simulink model "SynchGenerator_DQ_ThreePhaseFault"  (R2018a)
settings: Solver=FixedStepAuto  StartTime=0.0  StopTime=0.3  FixedStep=0.00005  MaxStep=200e-6  RelTol=1e-4  EnableMultiTasking=on
values from neighbouring files (symbols this model uses):
  fn = 60    [param_SynchGenerator_Kundur_3_1.m]    (also in param_SynchGenerator_Kundur_3_1_mathworks.m)
  ifn = 1300    [param_SynchGenerator_Kundur_3_1.m]    (also in param_SynchGenerator_Kundur_3_1_mathworks.m)
  Isbase = Pn/Vn/sqrt(3)*sqrt(2)    [param_SynchGenerator_Kundur_3_1.m]    (also in param_SynchGenerator_Kundur_3_1_mathworks.m)
  J = 2*H*Pn/wm^2    (= 28897.645918)    [param_SynchGenerator_Kundur_3_1.m]    (also in param_SynchGenerator_Kundur_3_1_mathworks.m)
  Ll = 0.4129e-3    (= 0.0004129)    [param_SynchGenerator_Kundur_3_1.m]    (also in param_SynchGenerator_Kundur_3_1_mathworks.m)
  Llfd = Llfd_pu*Lfbase    (= 0.0521181521186)    [param_SynchGenerator_Kundur_3_1.m]    (also in param_SynchGenerator_Kundur_3_1_mathworks.m)
  Llkd_pu = 0.1713    [param_SynchGenerator_Kundur_3_1.m]    (also in param_SynchGenerator_Kundur_3_1_mathworks.m)
  Llkq1_pu = 0.7252    [param_SynchGenerator_Kundur_3_1.m]    (also in param_SynchGenerator_Kundur_3_1_mathworks.m)
  Llkq2_pu = 0.125    [param_SynchGenerator_Kundur_3_1.m]    (also in param_SynchGenerator_Kundur_3_1_mathworks.m)
  Lmd = 4.5696e-3    (= 0.0045696)    [param_SynchGenerator_Kundur_3_1.m]    (also in param_SynchGenerator_Kundur_3_1_mathworks.m)
  Lmq = 4.432e-3    (= 0.004432)    [param_SynchGenerator_Kundur_3_1.m]    (also in param_SynchGenerator_Kundur_3_1_mathworks.m)
  Lsbase = Zsbase/wbase    (= 0.00275295036699)    [param_SynchGenerator_Kundur_3_1.m]    (also in param_SynchGenerator_Kundur_3_1_mathworks.m)
  Ns_Nf = 2/3*Ifbase/Isbase    [param_SynchGenerator_Kundur_3_1.m]    (also in param_SynchGenerator_Kundur_3_1_mathworks.m)
  Pn = 555e6    (= 555000000)    [param_SynchGenerator_Kundur_3_1.m]    (also in param_SynchGenerator_Kundur_3_1_mathworks.m)
  Rf = 0.0715    [param_SynchGenerator_Kundur_3_1.m]    (also in param_SynchGenerator_Kundur_3_1_mathworks.m)
  Rkd_pu = 0.0284    [param_SynchGenerator_Kundur_3_1.m]    (also in param_SynchGenerator_Kundur_3_1_mathworks.m)
  Rkq1_pu = 0.00619    [param_SynchGenerator_Kundur_3_1.m]    (also in param_SynchGenerator_Kundur_3_1_mathworks.m)
  Rkq2_pu = 0.02368    [param_SynchGenerator_Kundur_3_1.m]    (also in param_SynchGenerator_Kundur_3_1_mathworks.m)
  Rs = 0.0031    [param_SynchGenerator_Kundur_3_1.m]    (also in param_SynchGenerator_Kundur_3_1_mathworks.m)
  Vn = 24e3    (= 24000)    [param_SynchGenerator_Kundur_3_1.m]    (also in param_SynchGenerator_Kundur_3_1_mathworks.m)
  Vsbase = Vn/sqrt(3)*sqrt(2)    [param_SynchGenerator_Kundur_3_1.m]    (also in param_SynchGenerator_Kundur_3_1_mathworks.m)
  Zsbase = Vn^2/Pn    (= 1.03783783784)    [param_SynchGenerator_Kundur_3_1.m]    (also in param_SynchGenerator_Kundur_3_1_mathworks.m)
libraries: powerlib x9
Description:
  | Copyright 2008-2016 The MathWorks, Inc.
settings Model: Creator=MathWorks  LastModifiedBy=acs-mmi
settings DataIOCC: LimitDataPoints=on  SaveFormat=Array
settings OptimizationCC: ExpressionDepthLimit=2147483647  LifeSpan=inf
settings DebuggingCC: UnderspecifiedInitializationDetection=Classic  MergeDetectMultiDrivingBlocksExec=none  SolverPrmCheckMsg=warning  UnconnectedInputMsg=none  UnconnectedOutputMsg=none  UnconnectedLineMsg=none  StateNameClashWarn=warning  SFUnexpectedBacktrackingDiag=warning  SFNoUnconditionalDefaultTransitionDiag=warning  SFExecutionAtInitializationDiag=none
settings HardwareCC: ProdBitPerPointer=32  ProdBitPerSizeT=32  ProdBitPerPtrDiffT=32  ProdLargestAtomicFloat=None  ProdIntDivRoundTo=Undefined  ProdEndianess=Unspecified  ProdWordSize=32  ProdHWDeviceType=32-bit Generic
settings ModelReferenceCC: PropagateSignalLabelsOutOfModel=off
settings CodeAppCC: StateflowObjectComments=on
settings GRTTargetCC: TargetLangStandard=C89/C90 (ANSI)  GeneratePreprocessorConditionals=Disable all
settings ConfigComp: CovMetricSettings=dw  CovHtmlReporting=on  CovSaveCumulativeToWorkspaceVar=on  CovSaveSingleToWorkspaceVar=on  CovExternalEMLEnable=off  CovSFcnEnable=off
settings SimscapeCC: SimscapeNormalizeSystem=off

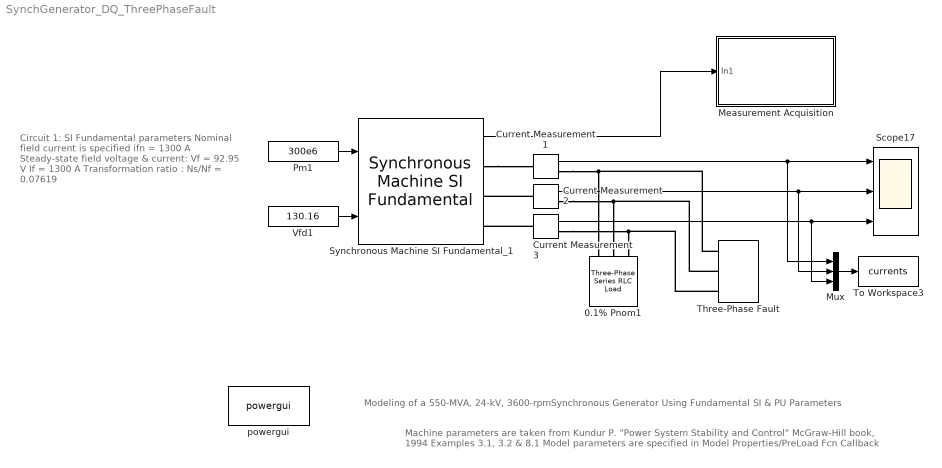
== system SynchGenerator_DQ_ThreePhaseFault ==
  note: Circuit 1: SI Fundamental parameters
      |
      | Nominal field current is specified
      |      ifn = 1300 A
      | Steady-state field voltage & current:
      |     Vf = 92.95 V
      |     If  = 1300 A
      | Transformation ratio :
      |     Ns/Nf = 0.07619
  note: Machine parameters are taken from Kundur P.  "Power System Stability and Control" McGraw-Hill  book, 1994 Examples 3.1, 3.2 &  8.1
      | Model parameters are specified  in Model Properties/PreLoad Fcn Callback
  note: Modeling of a 550-MVA, 24-kV, 3600-rpmSynchronous Generator Using Fundamental SI & PU Parameters
  0.1% Pnom1 : powerlib/Elements/Three-Phase Series RLC Load  LConnTagsString=A|B|C  Configuration=Y (grounded)  NominalVoltage=24e3  Vabc=[1e3 1e3 1e3]  Vabcp=[1e3 1e3 1e3]  NominalFrequency=60  UnbalancedPower=off  ActivePower=300e6  InductivePower=0  CapacitivePower=0  Pabc=[10e3 9e3 11e3]  QLabc=[100 90 110]  QCabc=[100 90 110]  Pabcp=[10e3 9e3 11e3]  QLabcp=[100 90 110]  QCabcp=[100 90 110]  Measurements=Branch voltages and currents  LoadType=constant Z
  Current Measurement1 : powerlib/Measurements/Current Measurement  PhasorSimulation=off  OutputType=Complex  PSBequivalent=0
  Current Measurement2 : powerlib/Measurements/Current Measurement  PhasorSimulation=off  OutputType=Complex  PSBequivalent=0
  Current Measurement3 : powerlib/Measurements/Current Measurement  PhasorSimulation=off  OutputType=Complex  PSBequivalent=0
  Measurement Acquisition : Subsystem
  Mux : Mux  Inputs=3
  Pm1 : Constant  Value=300e6
  Scope17 : Scope  NumInputPorts=3
  Synchronous Machine SI Fundamental_1 : powerlib/Machines/Synchronous Machine SI Fundamental  PresetModel=No  MechanicalLoad=Mechanical power Pm  ShowDetailedParameters=on  RotorType=Round  Units=SI fundamental parameters  MeasurementBus=off  NominalParameters="[ Pn  Vn    fn  ifn ]"  Stator="[ Rs    Ll    Lmd     Lmq ]"  Field="[Rf   Llfd ]*3/2*(Ns_Nf)^2"  Dampers2="[Rkd_pu Llkd_pu  Rkq1_pu  Llkq1_pu Rkq2_pu  Llkq2_pu ] .*[Zsbase  Lsbase  Zsbase  Lsbase  Zsbase  Lsbase]"  Dampers1="[Rkd_pu  Llkd_pu  Rkq1_pu  Llkq1_pu].*[Zsbase  Lsbase  Zsbase  Lsbase]"  Mechanical="[ J  0 1 ]"  PolePairs=1  InitialConditions=[0 -46.4745 10206.21 10206.21 10206.21 -180 -60 60 130.16]  SetSaturation=off  Saturation=[695.64,774.7,917.5,1001.6,1082.2,1175.9,1293.6,1430.2,1583.7;9660,10623,12243,13063,13757,14437,15180,15890,16567]  DisplayVfd=off  LoadFlowParameters=[4 300000000 0 0 0]  TsPowergui=0  TsBlock=-1  IterativeModel=Trapezoidal iterative (alg. loop)  IterativeDiscreteModel=Trapezoidal non iterative  BusType=swing  Pref=0  Qref=0  Qmin=-inf  Qmax=inf  PLF=0  QLF=0
      settings: SourceProductName=Simscape Power Systems  SourceProductBaseCode=PS
  Three-Phase Fault : powerlib/Elements/Three-Phase Fault  InitialStates=0  FaultA=on  FaultB=on  FaultC=on  GroundFault=on  SwitchTimes=[0.10005 0.2]  External=off  SwitchStatus=NaN  FaultResistance=0.001  GroundResistance=0.01  SnubberResistance=1e6  SnubberCapacitance=inf  Measurements=Fault voltages and currents
  To Workspace3 : ToWorkspace  VariableName=currents  SaveFormat=Timeseries  SampleTime=-1
  Vfd1 : Constant  Value=130.16
  powergui : powerlib/powergui  Priority=1  SimulationMode=Discrete  SampleTime=50e-6  frequency=60  Iterations=50  frequencyindice=60  Pbase=100e6  ErrMax=0.0001  UnitsV=kV  UnitsW=MW  buscounter=0  FunctionMessages=off  echomessages=off  EnableUseOfTLC=off  CurrentSourceSwitches=off  DisableSnubberDevices=off  DisableRonSwitches=off  DisableVfSwitches=off  DisplayEquations=off  SolverType=Tustin/Backward Euler (TBE)  Interpol=off  ExternalGateDelay=off  methode=off  Ts=100  x0status=blocks  SPID=off  SwTol=0  HookPort=off  RestoreLinks=warning  ResistiveCurrentMeasurement=off  Frange=[0:2:500]  Ylog=off  Xlog=on  ShowGrid=off  save=off  variable=ZData  structure=0  ZoomFFT=off  StartTime=0.0  cycles=1  DisplayStyle=1  fundamental=60  FreqAxis=off  MaxFrequency=1000  frequencyindicesteady=1  RmsSteady=1  display=off
  wires:
  Pm1/1 -> Synchronous Machine SI Fundamental_1/1
  Vfd1/1 -> Synchronous Machine SI Fundamental_1/2
  Current Measurement1/1 -> Mux/1, Scope17/1
  Current Measurement2/1 -> Mux/2, Scope17/2
  Current Measurement3/1 -> Mux/3, Scope17/3
  Mux/1 -> To Workspace3/1
  Synchronous Machine SI Fundamental_1/1 -> Measurement Acquisition/1(In1)
  connections:
  Three-Phase Fault/LConn3 -- Current Measurement3/RConn1 -- 0.1% Pnom1/LConn3
  Three-Phase Fault/LConn2 -- Current Measurement2/RConn1 -- 0.1% Pnom1/LConn2
  Synchronous Machine SI Fundamental_1/RConn1 -- Current Measurement1/LConn1
  Current Measurement1/RConn1 -- Three-Phase Fault/LConn1 -- 0.1% Pnom1/LConn1
  Current Measurement2/LConn1 -- Synchronous Machine SI Fundamental_1/RConn2
  Current Measurement3/LConn1 -- Synchronous Machine SI Fundamental_1/RConn3

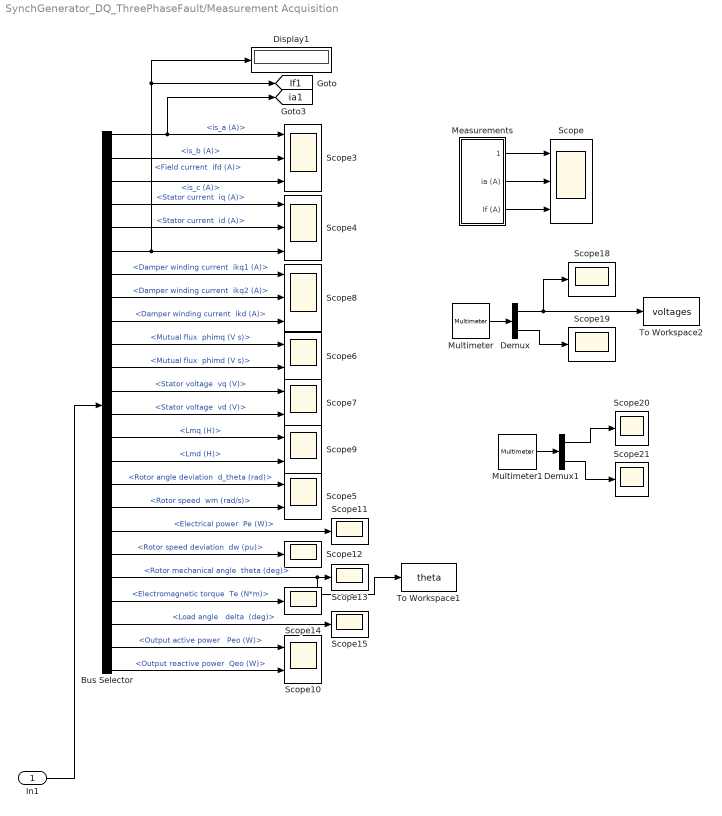
== system SynchGenerator_DQ_ThreePhaseFault/Measurement Acquisition ==
  In1 : Inport
  Bus Selector : BusSelector  OutputSignals="Stator current.is_a (A),Stator current.is_b (A),Stator current.is_c (A),dq0 components.Stator current  iq (A),dq0 components.Stator current  id (A),dq0 components.Field current  ifd (A),dq0 components.Damper winding current  ikq1 (A),dq0 components.Damper winding current  ikq2 (A),dq0 components.Damper winding current  ikd (A),dq0 components.Mutual flux  phimq (V s),dq0 components.Mutual flux  phimd (V s),dq0 components.Stator voltage  vq (V),dq0 components.Stator voltage  vd (V),dq0 components.Lmq (H),dq0 components.Lmd (H),Mechanical.Rotor angle deviation  d_theta (rad),Mechanical.Rotor speed  wm (rad/s),Mechanical.Electrical power  Pe (W),Mechanical.Rotor speed deviation  dw (pu),Mechanical.Rotor mechanical angle  theta (deg),Mechanical.Electromagnetic torque  Te (N*m),Load angle   delta  (deg),Output active power   Peo (W),Output reactive power  Qeo (W)"
  Demux : Demux  Outputs=2
  Demux1 : Demux  Outputs=2
  Display1 : Display
  Measurements : Subsystem
  Multimeter : powerlib/Measurements/Multimeter  PhasorSimulation=off  OutputType=Complex  sel=[1 2 3 7 8 9]  L=12  Gain=[1 1 1 1 1 1]  yselected={'Uag: 0.1% Pnom1','Ubg: 0.1% Pnom1','Ucg: 0.1% Pnom1','Iag: 0.1% Pnom1','Ibg: 0.1% Pnom1','Icg: 0.1% Pnom1'};  PSBOutputType=1  PSBequivalent=0  AxesSetting=[0,0.1,-100,100]  Display=0  SavedBlockNames=-11
  Multimeter1 : powerlib/Measurements/Multimeter  PhasorSimulation=off  OutputType=Complex  sel=[5 6 4 11 12 10]  L=12  Gain=[1 1 1 1 1 1]  yselected={'Ub: Three-Phase Fault/Fault A','Ub: Three-Phase Fault/Fault B','Ub: Three-Phase Fault/Fault C','Ib: Three-Phase Fault/Fault A','Ib: Three-Phase Fault/Fault B','Ib: Three-Phase Fault/Fault C'};  PSBOutputType=1  PSBequivalent=0  AxesSetting=[0,0.1,-100,100]  Display=0  SavedBlockNames=-11
  Scope{,3..4,8} (4 alike) : Scope  NumInputPorts=3
  Scope{5..7,9..10} (5 alike) : Scope  NumInputPorts=2
  Scope{11..15,18..21} (9 alike) : Scope
  To Workspace1 : ToWorkspace  VariableName=theta  SampleTime=-1
  To Workspace2 : ToWorkspace  VariableName=voltages  SaveFormat=Timeseries  SampleTime=-1
  tag scope: If1=global, ia1=global
  wires:
  Bus Selector/6 -> Scope4/3, Display1/1, [If1]  "<Field current  ifd (A)>"
  Demux/1 -> To Workspace2/1, Scope18/1
  Bus Selector/14 -> Scope9/1  "<Lmq (H)>"
  Bus Selector/23 -> Scope10/1  "<Output active power   Peo (W)>"
  Bus Selector/1 -> [ia1], Scope3/1  "<is_a (A)>"
  Measurements/3(If (A)) -> Scope/3
  Bus Selector/5 -> Scope4/2  "<Stator current  id (A)>"
  Bus Selector/16 -> Scope5/1  "<Rotor angle deviation  d_theta (rad)>"
  Bus Selector/7 -> Scope8/1  "<Damper winding current  ikq1 (A)>"
  Measurements/2(ia (A)) -> Scope/2
  Bus Selector/20 -> To Workspace1/1, Scope13/1  "<Rotor mechanical angle  theta (deg)>"
  Multimeter1/1 -> Demux1/1
  Bus Selector/3 -> Scope3/3  "<is_c (A)>"
  Bus Selector/4 -> Scope4/1  "<Stator current  iq (A)>"
  Bus Selector/24 -> Scope10/2  "<Output reactive power  Qeo (W)>"
  Bus Selector/2 -> Scope3/2  "<is_b (A)>"
  In1/1 -> Bus Selector/1
  Bus Selector/11 -> Scope6/2  "<Mutual flux  phimd (V s)>"
  Bus Selector/13 -> Scope7/2  "<Stator voltage  vd (V)>"
  Bus Selector/12 -> Scope7/1  "<Stator voltage  vq (V)>"
  Bus Selector/15 -> Scope9/2  "<Lmd (H)>"
  Bus Selector/8 -> Scope8/2  "<Damper winding current  ikq2 (A)>"
  Bus Selector/22 -> Scope15/1  "<Load angle   delta  (deg)>"
  Bus Selector/18 -> Scope11/1  "<Electrical power  Pe (W)>"
  Bus Selector/21 -> Scope14/1  "<Electromagnetic torque  Te (N*m)>"
  Measurements/1(Vab (pu)) -> Scope/1
  Multimeter/1 -> Demux/1
  Bus Selector/17 -> Scope5/2  "<Rotor speed  wm (rad/s)>"
  Demux1/2 -> Scope21/1
  Demux/2 -> Scope19/1
  Demux1/1 -> Scope20/1
  Bus Selector/19 -> Scope12/1  "<Rotor speed deviation  dw (pu)>"
  Bus Selector/10 -> Scope6/1  "<Mutual flux  phimq (V s)>"
  Bus Selector/9 -> Scope8/3  "<Damper winding current  ikd (A)>"

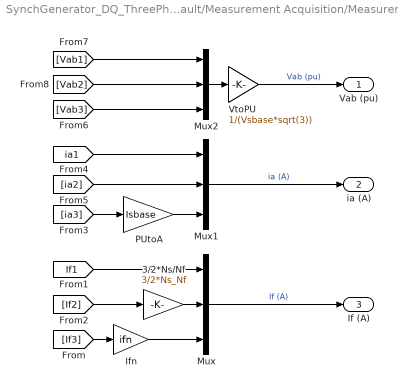
== system SynchGenerator_DQ_ThreePhaseFault/Measurement Acquisition/Measurements ==
  3/2*Ns/Nf : Gain  Gain=3/2*Ns_Nf
  Ifn : Gain  Gain=ifn
  Mux : Mux  Inputs=3
  Mux1 : Mux  Inputs=3
  Mux2 : Mux  Inputs=3
  PUtoA : Gain  Gain=Isbase
  VtoPU : Gain  Gain=1/(Vsbase*sqrt(3))
  Vab (pu) : Outport
  ia (A) : Outport  Port=2
  If (A) : Outport  Port=3
  wires:
  [Vab2] -> Mux2/2
  [Vab1] -> Mux2/1
  Mux2/1 -> VtoPU/1
  VtoPU/1 -> Vab (pu)/1  "Vab (pu)"
  [ia2] -> Mux1/2
  [Vab3] -> Mux2/3
  PUtoA/1 -> Mux1/3
  Ifn/1 -> Mux/3
  Mux/1 -> If (A)/1  "If (A)"
  [ia3] -> PUtoA/1
  [If3] -> Ifn/1
  [If2] -> 3/2*Ns/Nf/1
  Mux1/1 -> ia (A)/1  "ia (A)"
  3/2*Ns/Nf/1 -> Mux/2
  [If1] -> Mux/1
  [ia1] -> Mux1/1
